simulink model "allmodes"  (Simulink 7.4)
settings: Solver=ode23tb  StartTime=0.0  StopTime=inf  MaxStep=1e-4  RelTol=1e-4
undefined symbols (not defined in the file): Ion, Lithium
libraries: powerlib x185, electricdrivelib x21, powerlib_extras x19, simulink x5
(part 2 of 7)

== system allmodes/battery controller /SUIM1 ==
  Ibref-SUIM : Inport
  Add : Sum  OutDataType=fixdt(1, 16)  OutScaling=2^-10
  Add1 : Sum  Inputs=+-  OutDataType=fixdt(1, 16)  OutScaling=2^-10
  Gain1 : Gain  Gain=0.025  ParameterDataType=fixdt(1, 16)  ParameterScaling=2^0  OutDataType=fixdt(1, 16)  OutScaling=2^0
  Gain2 : Gain  Gain=0.8  ParameterDataType=fixdt(1, 16)  ParameterScaling=2^0  OutDataType=fixdt(1, 16)  OutScaling=2^0
  Integrator : Integrator
  Memory : Memory  X0=200
  Saturation : Saturate  UpperLimit=1  LowerLimit=-1  OutDataType=fixdt(1, 16)  OutScaling=2^0
  Saturation1 : Saturate  UpperLimit=1.01  LowerLimit=0.1  OutDataType=fixdt(1, 16)  OutScaling=2^0
  Subsystem : Subsystem
  Subsystem1 : Subsystem
  Subsystem2 : Subsystem
  Subsystem3 : Subsystem
  Sum : Sum  Inputs=|++  OutDataType=fixdt(1, 16)  OutScaling=2^0
  Sum10 : Sum  Inputs=++|  OutDataType=fixdt(1, 16)  OutScaling=2^0
  Sum2 : Sum  Inputs=|++  OutDataType=fixdt(1, 16)  OutScaling=2^0
  Sum{3..4,7..8} (4 alike) : Sum  Inputs=|+-  OutDataType=fixdt(1, 16)  OutScaling=2^0
  Sum5 : Sum  Inputs=|++  OutDataType=fixdt(1, 16)  OutScaling=2^0
  Sum6 : Sum  Inputs=+|+|+  OutDataType=fixdt(1, 16)  OutScaling=2^0
  Sum9 : Sum  Inputs=|+-+  OutDataType=fixdt(1, 16)  OutScaling=2^0
  Switch : Switch  Threshold=400*0.3  OutDataType=fixdt(1, 16)  OutScaling=2^0
  Switch1 : Switch  Threshold=99.999999  OutDataType=fixdt(1, 16)  OutScaling=2^0
  Switch2 : Switch  Threshold=99.999999  OutDataType=fixdt(1, 16)  OutScaling=2^0
  Transfer Fcn1 : TransferFcn  Numerator=1  Denominator=[1/(10) 1]
  Transport Delay : TransportDelay  DelayTime=2
  Transport Delay1 : TransportDelay  DelayTime=2
  ain1 : Gain  Gain=0.25  ParameterDataType=fixdt(1, 16)  ParameterScaling=2^0  OutDataType=fixdt(1, 16)  OutScaling=2^0
  ain2 : Gain  Gain=1/700  ParameterDataType=fixdt(1, 16)  ParameterScaling=2^0  OutDataType=fixdt(1, 16)  OutScaling=2^0
  ain3 : Gain  Gain=1/16.5  ParameterDataType=fixdt(1, 16)  ParameterScaling=2^0  OutDataType=fixdt(1, 16)  OutScaling=2^0
  ain4 : Gain  Gain=700  ParameterDataType=fixdt(1, 16)  ParameterScaling=2^0  OutDataType=fixdt(1, 16)  OutScaling=2^0
  ain5 : Gain  Gain=0.75  ParameterDataType=fixdt(1, 16)  ParameterScaling=2^0  OutDataType=fixdt(1, 16)  OutScaling=2^0
  ain6 : Gain  Gain=16.5  ParameterDataType=fixdt(1, 16)  ParameterScaling=2^0  OutDataType=fixdt(1, 16)  OutScaling=2^0
  ain7 : Gain  Gain=0.03  ParameterDataType=fixdt(1, 16)  ParameterScaling=2^0  OutDataType=fixdt(1, 16)  OutScaling=2^0
  ain8 : Gain  Gain=7  ParameterDataType=fixdt(1, 16)  ParameterScaling=2^0  OutDataType=fixdt(1, 16)  OutScaling=2^0
  ain9 : Gain  Gain=0.3  ParameterDataType=fixdt(1, 16)  ParameterScaling=2^0  OutDataType=fixdt(1, 16)  OutScaling=2^0
  tag scope: Ibrefs=global, boost=global, buck=global
  wires:
  Sum4/1 -> ain1/1, Subsystem2/1(In1)
  ain2/1 -> Saturation/1
  Subsystem2/1(Out1) -> Sum2/1
  ain1/1 -> Sum2/2
  Saturation/1 -> ain4/1, Switch1/3
  ain4/1 -> Sum3/1
  Sum3/1 -> ain3/1
  Subsystem1/1(Out1) -> Sum6/2
  ain5/1 -> Sum6/3
  Sum7/1 -> ain5/1, Subsystem1/1(In1)
  Sum2/1 -> Sum5/1
  Sum5/1 -> Sum8/1
  Sum8/1 -> ain6/1, Sum10/2
  Subsystem3/1(Out1) -> Sum/1
  ain6/1 -> Sum/2
  Sum/1 -> Sum9/1
  Sum9/1 -> Sum3/2, ain2/1
  ain3/1 -> Sum10/1
  ain7/1 -> Sum9/2
  Sum6/1 -> Sum4/1
  Sum10/1 -> Subsystem3/1(In1)
  [VcSUIM] -> Sum4/2
  [VcSUIM] -> Sum9/3
  [IbSUIM] -> Sum7/2
  [IbSUIM] -> Sum5/2
  [VbSUIM] -> Sum6/1
  [ISUIM] -> ain7/1
  [ISUIM] -> Sum8/2
  Subsystem/2(Out2) -> [boost]
  Subsystem/1(Out1) -> [buck]
  Transfer Fcn1/1 -> Sum7/1, [Ibrefs]
  [ts] -> Subsystem/Enable
  [VbSUIM] -> Switch/2
  ain8/1 -> Switch/1
  ain9/1 -> Switch/3
  Ibref-SUIM/1 -> ain8/1, ain9/1
  Switch/1 -> Transfer Fcn1/1
  [VbSUIM] -> Add1/2
  Add1/1 -> Gain1/1, Gain2/1
  [VbSUIM] -> Switch2/3
  [soc] -> Transport Delay1/1
  Transport Delay1/1 -> Switch2/2
  Add/1 -> Saturation1/1
  Gain1/1 -> Add/2
  Integrator/1 -> Add/1
  Gain2/1 -> Integrator/1
  Switch2/1 -> Add1/1, Memory/1
  Memory/1 -> Switch2/1
  Switch1/1 -> Subsystem/1(In1)
  [soc] -> Transport Delay/1
  Saturation1/1 -> Switch1/1
  Transport Delay/1 -> Switch1/2

== system allmodes/battery controller /mode selector ==
  In1 : Inport
  Constant33 : Constant  Value=[0 1 0 0 0 0 0 0 0 0 0 0 0 0 0 0 0 0 0 0 0]  OutDataType=fixdt(1, 16)  OutScaling=2^0
  Constant34 : Constant  Value=[0 1 1 1 1 0 0 0 0 0 0 0 0 0 0 0 0 0 0 0 0]  OutDataType=fixdt(1, 16)  OutScaling=2^0
  Constant35 : Constant  Value=[0 1 1 1 1 1 1 0 0 0 0 0 0 0 0 0 0 0 0 0 0]  OutDataType=fixdt(1, 16)  OutScaling=2^0
  Constant36 : Constant  Value=[0 1 1 1 1 1 1 1 1 1 1 1 1 0 0 0 0 0 0 0 0]  OutDataType=fixdt(1, 16)  OutScaling=2^0
  Constant37 : Constant  Value=[0 1 1 1 1 1 1 1 1 1 1 1 1 1 1 1 1 1 1 1 1]  OutDataType=fixdt(1, 16)  OutScaling=2^0
  Constant38 : Constant  Value=[0 1 1 0 0 0 0 0 0 0 0 0 0 0 0 0 0 0 0 0 0]  OutDataType=fixdt(1, 16)  OutScaling=2^0
  Constant39 : Constant  Value=[0 1 1 1 1 0 0 0 0 0 0 0 0 0 0 0 0 0 0 0 0]  OutDataType=fixdt(1, 16)  OutScaling=2^0
  Constant40 : Constant  Value=[0 1 1 1 1 1 1 1 1 0 0 0 0 0 0 0 0 0 0 0 0]  OutDataType=fixdt(1, 16)  OutScaling=2^0
  Constant41 : Constant  Value=[0 1 1 1 1 1 1 1 1 1 1 1 1 1 1 1 1 0 0 0 0]  OutDataType=fixdt(1, 16)  OutScaling=2^0
  Constant42 : Constant  Value=[0 1 1 1 1 1 1 1 1 1 1 0 0 0 0 0 0 0 0 0 0]  OutDataType=fixdt(1, 16)  OutScaling=2^0
  Constant43 : Constant  Value=[1 1 1 1 1 1 1 1 1 1 1 1 1 1 1 1 1 1 1 1 1]  OutDataType=fixdt(1, 16)  OutScaling=2^0
  Constant44 : Constant  Value=[0 1 1 0 0 0 0 0 0 0 0 0 0 0 0 0 0 0 0 0 0]  OutDataType=fixdt(1, 16)  OutScaling=2^0
  Constant45 : Constant  Value=[0 1 1 1 1 1 1 1 1 1 1 1 1 1 1 1 1 1 1 1 1]  OutDataType=fixdt(1, 16)  OutScaling=2^0
  Constant46 : Constant  Value=[0 1 1 1 1 1 1 1 1 1 1 0 0 0 0 0 0 0 0 0 0]  OutDataType=fixdt(1, 16)  OutScaling=2^0
  Constant47 : Constant  Value=[0 1 1 1 1 1 1 1 1 1 1 0 0 0 0 0 0 0 0 0 0]  OutDataType=fixdt(1, 16)  OutScaling=2^0
  Constant48 : Constant  Value=[0 1 1 1 1 1 1 1 1 1 1 1 1 1 1 1 1 1 1 1 1]  OutDataType=fixdt(1, 16)  OutScaling=2^0
  Constant{49..52} (4 alike) : Constant  Value=[1 0 0 0 0 0 0 0 0 0 0 0 0 0 0 0 0 0 0 0 0]  OutDataType=fixdt(1, 16)  OutScaling=2^0
  Constant53 : Constant  Value=[0 1 0 0 0 0 0 0 0 0 0 0 0 0 0 0 0 0 0 0 0]  OutDataType=fixdt(1, 16)  OutScaling=2^0
  Demux : Demux  Outputs=21
  Multiport Switch : MultiPortSwitch  Inputs=21  OutDataType=fixdt(1, 16)  OutScaling=2^0
  tag scope: ts=global, tv10=global, tv11=global, tv12=global, tv13=global, tv14=global, tv15=global, tv16=global, tv17=global, tv18=global, tv19=global, tv1=global, tv20=global, tv2=global, tv3=global, tv4=global, tv5=global, tv6=global, tv7=global, tv8=global, tv9=global
  wires:
  Constant33/1 -> Multiport Switch/2
  Constant44/1 -> Multiport Switch/3
  Constant47/1 -> Multiport Switch/4
  Constant48/1 -> Multiport Switch/5
  Constant49/1 -> Multiport Switch/6
  Constant50/1 -> Multiport Switch/7
  Constant51/1 -> Multiport Switch/8
  Constant52/1 -> Multiport Switch/9
  Constant53/1 -> Multiport Switch/10
  Constant34/1 -> Multiport Switch/11
  Constant35/1 -> Multiport Switch/12
  Constant36/1 -> Multiport Switch/13
  Constant37/1 -> Multiport Switch/14
  Multiport Switch/1 -> Demux/1
  Constant38/1 -> Multiport Switch/15
  Constant39/1 -> Multiport Switch/16
  Constant40/1 -> Multiport Switch/17
  Constant41/1 -> Multiport Switch/18
  Constant42/1 -> Multiport Switch/19
  Constant43/1 -> Multiport Switch/22
  Constant45/1 -> Multiport Switch/21
  Constant46/1 -> Multiport Switch/20
  Demux/1 -> [ts]
  Demux/2 -> [tv1]
  Demux/3 -> [tv2]
  Demux/4 -> [tv3]
  Demux/5 -> [tv4]
  Demux/6 -> [tv5]
  Demux/7 -> [tv6]
  Demux/8 -> [tv7]
  Demux/9 -> [tv8]
  Demux/10 -> [tv9]
  Demux/11 -> [tv10]
  Demux/12 -> [tv11]
  Demux/13 -> [tv12]
  Demux/14 -> [tv13]
  Demux/15 -> [tv14]
  Demux/16 -> [tv15]
  Demux/17 -> [tv16]
  Demux/18 -> [tv17]
  Demux/19 -> [tv18]
  Demux/20 -> [tv19]
  Demux/21 -> [tv20]
  In1/1 -> Multiport Switch/1

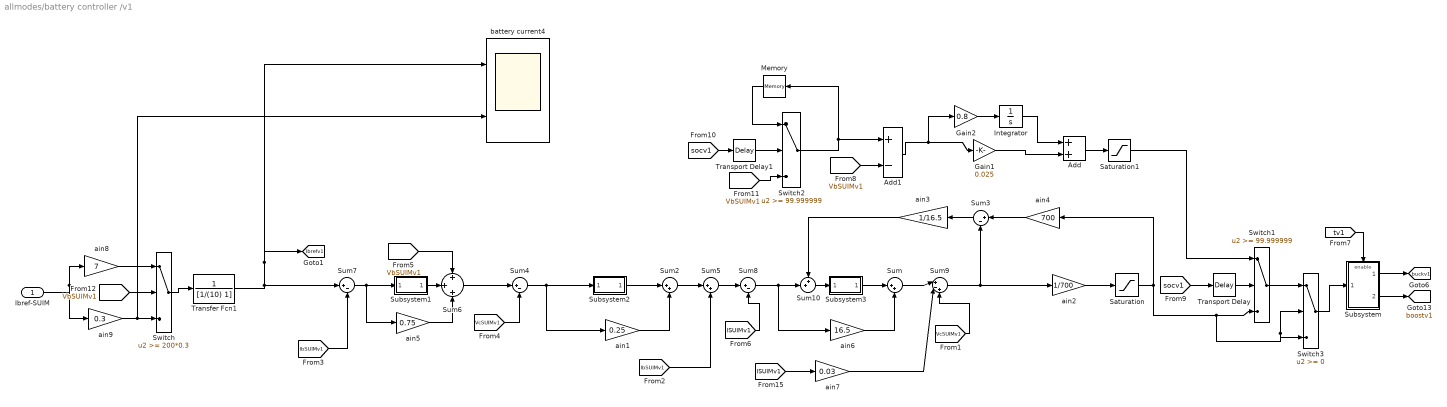
== system allmodes/battery controller /v1 ==
  Ibref-SUIM : Inport
  Add : Sum  OutDataType=fixdt(1, 16)  OutScaling=2^-10
  Add1 : Sum  Inputs=+-  OutDataType=fixdt(1, 16)  OutScaling=2^-10
  Gain1 : Gain  Gain=0.025  ParameterDataType=fixdt(1, 16)  ParameterScaling=2^0  OutDataType=fixdt(1, 16)  OutScaling=2^0
  Gain2 : Gain  Gain=0.8  ParameterDataType=fixdt(1, 16)  ParameterScaling=2^0  OutDataType=fixdt(1, 16)  OutScaling=2^0
  Integrator : Integrator
  Memory : Memory  X0=200
  Saturation : Saturate  UpperLimit=1  LowerLimit=-1  OutDataType=fixdt(1, 16)  OutScaling=2^0
  Saturation1 : Saturate  UpperLimit=1.01  LowerLimit=0.1  OutDataType=fixdt(1, 16)  OutScaling=2^0
  Subsystem : Subsystem
  Subsystem1 : Subsystem
  Subsystem2 : Subsystem
  Subsystem3 : Subsystem
  Sum : Sum  Inputs=|++  OutDataType=fixdt(1, 16)  OutScaling=2^0
  Sum10 : Sum  Inputs=++|  OutDataType=fixdt(1, 16)  OutScaling=2^0
  Sum2 : Sum  Inputs=|++  OutDataType=fixdt(1, 16)  OutScaling=2^0
  Sum{3..4,7..8} (4 alike) : Sum  Inputs=|+-  OutDataType=fixdt(1, 16)  OutScaling=2^0
  Sum5 : Sum  Inputs=|++  OutDataType=fixdt(1, 16)  OutScaling=2^0
  Sum6 : Sum  Inputs=+|+|+  OutDataType=fixdt(1, 16)  OutScaling=2^0
  Sum9 : Sum  Inputs=|+-+  OutDataType=fixdt(1, 16)  OutScaling=2^0
  Switch : Switch  Threshold=200*0.3  OutDataType=fixdt(1, 16)  OutScaling=2^0
  Switch1 : Switch  Threshold=99.999999  OutDataType=fixdt(1, 16)  OutScaling=2^0
  Switch2 : Switch  Threshold=99.999999  OutDataType=fixdt(1, 16)  OutScaling=2^0
  Switch3 : Switch  OutDataType=fixdt(1, 16)  OutScaling=2^0
  Transfer Fcn1 : TransferFcn  Numerator=1  Denominator=[1/(10) 1]
  Transport Delay : TransportDelay  DelayTime=2
  Transport Delay1 : TransportDelay  DelayTime=2
  ain1 : Gain  Gain=0.25  ParameterDataType=fixdt(1, 16)  ParameterScaling=2^0  OutDataType=fixdt(1, 16)  OutScaling=2^0
  ain2 : Gain  Gain=1/700  ParameterDataType=fixdt(1, 16)  ParameterScaling=2^0  OutDataType=fixdt(1, 16)  OutScaling=2^0
  ain3 : Gain  Gain=1/16.5  ParameterDataType=fixdt(1, 16)  ParameterScaling=2^0  OutDataType=fixdt(1, 16)  OutScaling=2^0
  ain4 : Gain  Gain=700  ParameterDataType=fixdt(1, 16)  ParameterScaling=2^0  OutDataType=fixdt(1, 16)  OutScaling=2^0
  ain5 : Gain  Gain=0.75  ParameterDataType=fixdt(1, 16)  ParameterScaling=2^0  OutDataType=fixdt(1, 16)  OutScaling=2^0
  ain6 : Gain  Gain=16.5  ParameterDataType=fixdt(1, 16)  ParameterScaling=2^0  OutDataType=fixdt(1, 16)  OutScaling=2^0
  ain7 : Gain  Gain=0.03  ParameterDataType=fixdt(1, 16)  ParameterScaling=2^0  OutDataType=fixdt(1, 16)  OutScaling=2^0
  ain8 : Gain  Gain=7  ParameterDataType=fixdt(1, 16)  ParameterScaling=2^0  OutDataType=fixdt(1, 16)  OutScaling=2^0
  ain9 : Gain  Gain=0.3  ParameterDataType=fixdt(1, 16)  ParameterScaling=2^0  OutDataType=fixdt(1, 16)  OutScaling=2^0
  battery current4 : Scope  NumInputPorts=2
      settings: TimeRange=0.25  YMin=460~30  YMax=660~30  SaveName=ScopeData7
  tag scope: Ibrefv1=global, boostv1=global, buckv1=global
  wires:
  Transfer Fcn1/1 -> Sum7/1, [Ibrefv1], battery current4/1
  Subsystem/1(Out1) -> [buckv1]
  Subsystem/2(Out2) -> [boostv1]
  [ISUIMv1] -> Sum8/2
  [ISUIMv1] -> ain7/1
  [VbSUIMv1] -> Sum6/1
  [IbSUIMv1] -> Sum5/2
  [IbSUIMv1] -> Sum7/2
  [VcSUIMv1] -> Sum9/3
  [VcSUIMv1] -> Sum4/2
  Sum10/1 -> Subsystem3/1(In1)
  Sum6/1 -> Sum4/1
  ain7/1 -> Sum9/2
  ain3/1 -> Sum10/1
  Sum9/1 -> ain2/1, Sum3/2
  Sum/1 -> Sum9/1
  ain6/1 -> Sum/2
  Subsystem3/1(Out1) -> Sum/1
  Sum8/1 -> Sum10/2, ain6/1
  Sum5/1 -> Sum8/1
  Sum2/1 -> Sum5/1
  Sum7/1 -> Subsystem1/1(In1), ain5/1
  ain5/1 -> Sum6/3
  Subsystem1/1(Out1) -> Sum6/2
  Sum3/1 -> ain3/1
  ain4/1 -> Sum3/1
  Saturation/1 -> ain4/1, Switch1/3, Switch3/3, Switch3/2
  ain1/1 -> Sum2/2
  Subsystem2/1(Out1) -> Sum2/1
  ain2/1 -> Saturation/1
  Sum4/1 -> Subsystem2/1(In1), ain1/1
  [tv1] -> Subsystem/Enable
  [VbSUIMv1] -> Add1/2
  Add1/1 -> Gain1/1, Gain2/1
  [VbSUIMv1] -> Switch2/3
  [socv1] -> Transport Delay1/1
  Transport Delay1/1 -> Switch2/2
  Add/1 -> Saturation1/1
  Gain1/1 -> Add/2
  Integrator/1 -> Add/1
  Gain2/1 -> Integrator/1
  Switch2/1 -> Add1/1, Memory/1
  Memory/1 -> Switch2/1
  [socv1] -> Transport Delay/1
  Transport Delay/1 -> Switch1/2
  Saturation1/1 -> Switch1/1
  [VbSUIMv1] -> Switch/2
  ain8/1 -> Switch/1
  ain9/1 -> Switch/3, battery current4/2
  Switch/1 -> Transfer Fcn1/1
  Ibref-SUIM/1 -> ain8/1, ain9/1
  Switch1/1 -> Switch3/1
  Switch3/1 -> Subsystem/1(In1)

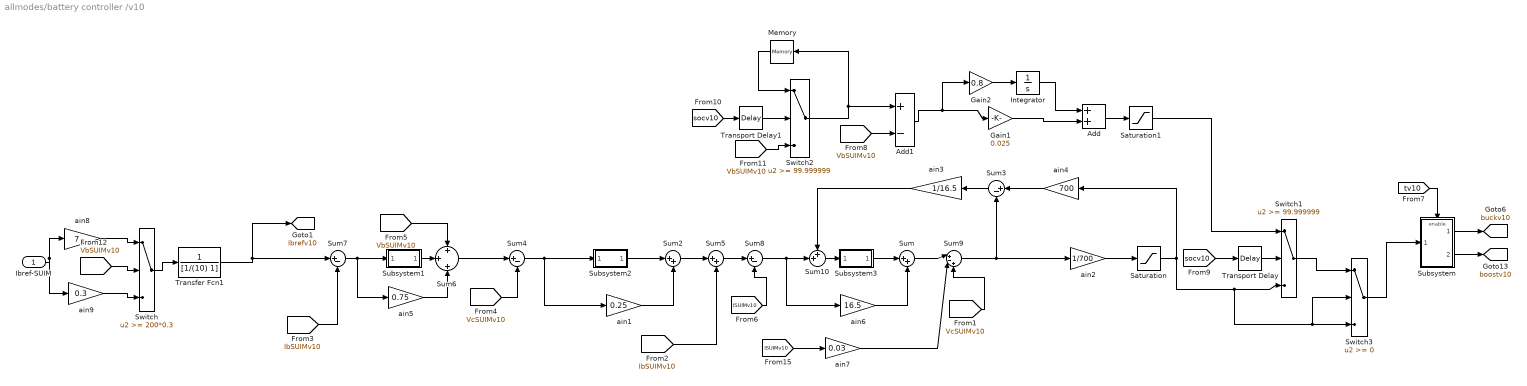
== system allmodes/battery controller /v10 ==
  Ibref-SUIM : Inport
  Add : Sum  OutDataType=fixdt(1, 16)  OutScaling=2^-10
  Add1 : Sum  Inputs=+-  OutDataType=fixdt(1, 16)  OutScaling=2^-10
  Gain1 : Gain  Gain=0.025  ParameterDataType=fixdt(1, 16)  ParameterScaling=2^0  OutDataType=fixdt(1, 16)  OutScaling=2^0
  Gain2 : Gain  Gain=0.8  ParameterDataType=fixdt(1, 16)  ParameterScaling=2^0  OutDataType=fixdt(1, 16)  OutScaling=2^0
  Integrator : Integrator
  Memory : Memory  X0=200
  Saturation : Saturate  UpperLimit=1  LowerLimit=-1  OutDataType=fixdt(1, 16)  OutScaling=2^0
  Saturation1 : Saturate  UpperLimit=1.01  LowerLimit=0.1  OutDataType=fixdt(1, 16)  OutScaling=2^0
  Subsystem : Subsystem
  Subsystem1 : Subsystem
  Subsystem2 : Subsystem
  Subsystem3 : Subsystem
  Sum : Sum  Inputs=|++  OutDataType=fixdt(1, 16)  OutScaling=2^0
  Sum10 : Sum  Inputs=++|  OutDataType=fixdt(1, 16)  OutScaling=2^0
  Sum2 : Sum  Inputs=|++  OutDataType=fixdt(1, 16)  OutScaling=2^0
  Sum{3..4,7..8} (4 alike) : Sum  Inputs=|+-  OutDataType=fixdt(1, 16)  OutScaling=2^0
  Sum5 : Sum  Inputs=|++  OutDataType=fixdt(1, 16)  OutScaling=2^0
  Sum6 : Sum  Inputs=+|+|+  OutDataType=fixdt(1, 16)  OutScaling=2^0
  Sum9 : Sum  Inputs=|+-+  OutDataType=fixdt(1, 16)  OutScaling=2^0
  Switch : Switch  Threshold=200*0.3  OutDataType=fixdt(1, 16)  OutScaling=2^0
  Switch1 : Switch  Threshold=99.999999  OutDataType=fixdt(1, 16)  OutScaling=2^0
  Switch2 : Switch  Threshold=99.999999  OutDataType=fixdt(1, 16)  OutScaling=2^0
  Switch3 : Switch  OutDataType=fixdt(1, 16)  OutScaling=2^0
  Transfer Fcn1 : TransferFcn  Numerator=1  Denominator=[1/(10) 1]
  Transport Delay : TransportDelay  DelayTime=2
  Transport Delay1 : TransportDelay  DelayTime=2
  ain1 : Gain  Gain=0.25  ParameterDataType=fixdt(1, 16)  ParameterScaling=2^0  OutDataType=fixdt(1, 16)  OutScaling=2^0
  ain2 : Gain  Gain=1/700  ParameterDataType=fixdt(1, 16)  ParameterScaling=2^0  OutDataType=fixdt(1, 16)  OutScaling=2^0
  ain3 : Gain  Gain=1/16.5  ParameterDataType=fixdt(1, 16)  ParameterScaling=2^0  OutDataType=fixdt(1, 16)  OutScaling=2^0
  ain4 : Gain  Gain=700  ParameterDataType=fixdt(1, 16)  ParameterScaling=2^0  OutDataType=fixdt(1, 16)  OutScaling=2^0
  ain5 : Gain  Gain=0.75  ParameterDataType=fixdt(1, 16)  ParameterScaling=2^0  OutDataType=fixdt(1, 16)  OutScaling=2^0
  ain6 : Gain  Gain=16.5  ParameterDataType=fixdt(1, 16)  ParameterScaling=2^0  OutDataType=fixdt(1, 16)  OutScaling=2^0
  ain7 : Gain  Gain=0.03  ParameterDataType=fixdt(1, 16)  ParameterScaling=2^0  OutDataType=fixdt(1, 16)  OutScaling=2^0
  ain8 : Gain  Gain=7  ParameterDataType=fixdt(1, 16)  ParameterScaling=2^0  OutDataType=fixdt(1, 16)  OutScaling=2^0
  ain9 : Gain  Gain=0.3  ParameterDataType=fixdt(1, 16)  ParameterScaling=2^0  OutDataType=fixdt(1, 16)  OutScaling=2^0
  tag scope: Ibrefv10=global, boostv10=global, buckv10=global
  wires:
  Ibref-SUIM/1 -> ain9/1, ain8/1
  Switch/1 -> Transfer Fcn1/1
  ain9/1 -> Switch/3
  ain8/1 -> Switch/1
  [VbSUIMv10] -> Switch/2
  Saturation1/1 -> Switch1/1
  Transport Delay/1 -> Switch1/2
  [socv10] -> Transport Delay/1
  Memory/1 -> Switch2/1
  Switch2/1 -> Memory/1, Add1/1
  Gain2/1 -> Integrator/1
  Integrator/1 -> Add/1
  Gain1/1 -> Add/2
  Add/1 -> Saturation1/1
  Transport Delay1/1 -> Switch2/2
  [socv10] -> Transport Delay1/1
  [VbSUIMv10] -> Switch2/3
  Add1/1 -> Gain2/1, Gain1/1
  [VbSUIMv10] -> Add1/2
  [tv10] -> Subsystem/Enable
  Sum4/1 -> ain1/1, Subsystem2/1(In1)
  ain2/1 -> Saturation/1
  Subsystem2/1(Out1) -> Sum2/1
  ain1/1 -> Sum2/2
  Saturation/1 -> ain4/1, Switch1/3, Switch3/3, Switch3/2
  ain4/1 -> Sum3/1
  Sum3/1 -> ain3/1
  Subsystem1/1(Out1) -> Sum6/2
  ain5/1 -> Sum6/3
  Sum7/1 -> ain5/1, Subsystem1/1(In1)
  Sum2/1 -> Sum5/1
  Sum5/1 -> Sum8/1
  Sum8/1 -> ain6/1, Sum10/2
  Subsystem3/1(Out1) -> Sum/1
  ain6/1 -> Sum/2
  Sum/1 -> Sum9/1
  Sum9/1 -> Sum3/2, ain2/1
  ain3/1 -> Sum10/1
  ain7/1 -> Sum9/2
  Sum6/1 -> Sum4/1
  Sum10/1 -> Subsystem3/1(In1)
  [VcSUIMv10] -> Sum4/2
  [VcSUIMv10] -> Sum9/3
  [IbSUIMv10] -> Sum7/2
  [IbSUIMv10] -> Sum5/2
  [VbSUIMv10] -> Sum6/1
  [ISUIMv10] -> ain7/1
  [ISUIMv10] -> Sum8/2
  Subsystem/2(Out2) -> [boostv10]
  Subsystem/1(Out1) -> [buckv10]
  Transfer Fcn1/1 -> [Ibrefv10], Sum7/1
  Switch1/1 -> Switch3/1
  Switch3/1 -> Subsystem/1(In1)

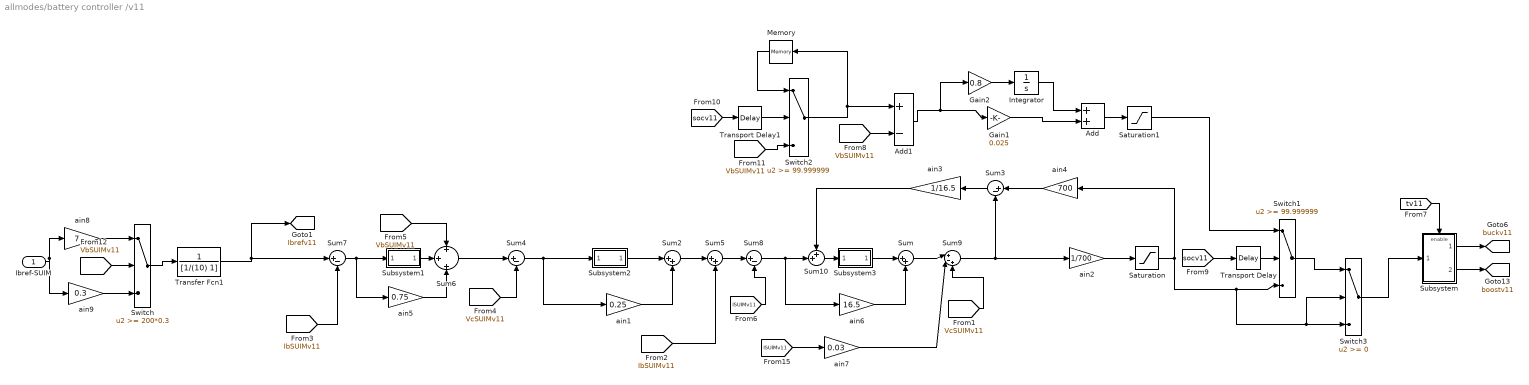
== system allmodes/battery controller /v11 ==
  Ibref-SUIM : Inport
  Add : Sum  OutDataType=fixdt(1, 16)  OutScaling=2^-10
  Add1 : Sum  Inputs=+-  OutDataType=fixdt(1, 16)  OutScaling=2^-10
  Gain1 : Gain  Gain=0.025  ParameterDataType=fixdt(1, 16)  ParameterScaling=2^0  OutDataType=fixdt(1, 16)  OutScaling=2^0
  Gain2 : Gain  Gain=0.8  ParameterDataType=fixdt(1, 16)  ParameterScaling=2^0  OutDataType=fixdt(1, 16)  OutScaling=2^0
  Integrator : Integrator
  Memory : Memory  X0=200
  Saturation : Saturate  UpperLimit=1  LowerLimit=-1  OutDataType=fixdt(1, 16)  OutScaling=2^0
  Saturation1 : Saturate  UpperLimit=1.01  LowerLimit=0.1  OutDataType=fixdt(1, 16)  OutScaling=2^0
  Subsystem : Subsystem
  Subsystem1 : Subsystem
  Subsystem2 : Subsystem
  Subsystem3 : Subsystem
  Sum : Sum  Inputs=|++  OutDataType=fixdt(1, 16)  OutScaling=2^0
  Sum10 : Sum  Inputs=++|  OutDataType=fixdt(1, 16)  OutScaling=2^0
  Sum2 : Sum  Inputs=|++  OutDataType=fixdt(1, 16)  OutScaling=2^0
  Sum{3..4,7..8} (4 alike) : Sum  Inputs=|+-  OutDataType=fixdt(1, 16)  OutScaling=2^0
  Sum5 : Sum  Inputs=|++  OutDataType=fixdt(1, 16)  OutScaling=2^0
  Sum6 : Sum  Inputs=+|+|+  OutDataType=fixdt(1, 16)  OutScaling=2^0
  Sum9 : Sum  Inputs=|+-+  OutDataType=fixdt(1, 16)  OutScaling=2^0
  Switch : Switch  Threshold=200*0.3  OutDataType=fixdt(1, 16)  OutScaling=2^0
  Switch1 : Switch  Threshold=99.999999  OutDataType=fixdt(1, 16)  OutScaling=2^0
  Switch2 : Switch  Threshold=99.999999  OutDataType=fixdt(1, 16)  OutScaling=2^0
  Switch3 : Switch  OutDataType=fixdt(1, 16)  OutScaling=2^0
  Transfer Fcn1 : TransferFcn  Numerator=1  Denominator=[1/(10) 1]
  Transport Delay : TransportDelay  DelayTime=2
  Transport Delay1 : TransportDelay  DelayTime=2
  ain1 : Gain  Gain=0.25  ParameterDataType=fixdt(1, 16)  ParameterScaling=2^0  OutDataType=fixdt(1, 16)  OutScaling=2^0
  ain2 : Gain  Gain=1/700  ParameterDataType=fixdt(1, 16)  ParameterScaling=2^0  OutDataType=fixdt(1, 16)  OutScaling=2^0
  ain3 : Gain  Gain=1/16.5  ParameterDataType=fixdt(1, 16)  ParameterScaling=2^0  OutDataType=fixdt(1, 16)  OutScaling=2^0
  ain4 : Gain  Gain=700  ParameterDataType=fixdt(1, 16)  ParameterScaling=2^0  OutDataType=fixdt(1, 16)  OutScaling=2^0
  ain5 : Gain  Gain=0.75  ParameterDataType=fixdt(1, 16)  ParameterScaling=2^0  OutDataType=fixdt(1, 16)  OutScaling=2^0
  ain6 : Gain  Gain=16.5  ParameterDataType=fixdt(1, 16)  ParameterScaling=2^0  OutDataType=fixdt(1, 16)  OutScaling=2^0
  ain7 : Gain  Gain=0.03  ParameterDataType=fixdt(1, 16)  ParameterScaling=2^0  OutDataType=fixdt(1, 16)  OutScaling=2^0
  ain8 : Gain  Gain=7  ParameterDataType=fixdt(1, 16)  ParameterScaling=2^0  OutDataType=fixdt(1, 16)  OutScaling=2^0
  ain9 : Gain  Gain=0.3  ParameterDataType=fixdt(1, 16)  ParameterScaling=2^0  OutDataType=fixdt(1, 16)  OutScaling=2^0
  tag scope: Ibrefv11=global, boostv11=global, buckv11=global
  wires:
  Ibref-SUIM/1 -> ain9/1, ain8/1
  Switch/1 -> Transfer Fcn1/1
  ain9/1 -> Switch/3
  ain8/1 -> Switch/1
  [VbSUIMv11] -> Switch/2
  Saturation1/1 -> Switch1/1
  Transport Delay/1 -> Switch1/2
  [socv11] -> Transport Delay/1
  Memory/1 -> Switch2/1
  Switch2/1 -> Memory/1, Add1/1
  Gain2/1 -> Integrator/1
  Integrator/1 -> Add/1
  Gain1/1 -> Add/2
  Add/1 -> Saturation1/1
  Transport Delay1/1 -> Switch2/2
  [socv11] -> Transport Delay1/1
  [VbSUIMv11] -> Switch2/3
  Add1/1 -> Gain2/1, Gain1/1
  [VbSUIMv11] -> Add1/2
  [tv11] -> Subsystem/Enable
  Sum4/1 -> ain1/1, Subsystem2/1(In1)
  ain2/1 -> Saturation/1
  Subsystem2/1(Out1) -> Sum2/1
  ain1/1 -> Sum2/2
  Saturation/1 -> ain4/1, Switch1/3, Switch3/3, Switch3/2
  ain4/1 -> Sum3/1
  Sum3/1 -> ain3/1
  Subsystem1/1(Out1) -> Sum6/2
  ain5/1 -> Sum6/3
  Sum7/1 -> ain5/1, Subsystem1/1(In1)
  Sum2/1 -> Sum5/1
  Sum5/1 -> Sum8/1
  Sum8/1 -> ain6/1, Sum10/2
  Subsystem3/1(Out1) -> Sum/1
  ain6/1 -> Sum/2
  Sum/1 -> Sum9/1
  Sum9/1 -> Sum3/2, ain2/1
  ain3/1 -> Sum10/1
  ain7/1 -> Sum9/2
  Sum6/1 -> Sum4/1
  Sum10/1 -> Subsystem3/1(In1)
  [VcSUIMv11] -> Sum4/2
  [VcSUIMv11] -> Sum9/3
  [IbSUIMv11] -> Sum7/2
  [IbSUIMv11] -> Sum5/2
  [VbSUIMv11] -> Sum6/1
  [ISUIMv11] -> ain7/1
  [ISUIMv11] -> Sum8/2
  Subsystem/2(Out2) -> [boostv11]
  Subsystem/1(Out1) -> [buckv11]
  Transfer Fcn1/1 -> [Ibrefv11], Sum7/1
  Switch1/1 -> Switch3/1
  Switch3/1 -> Subsystem/1(In1)

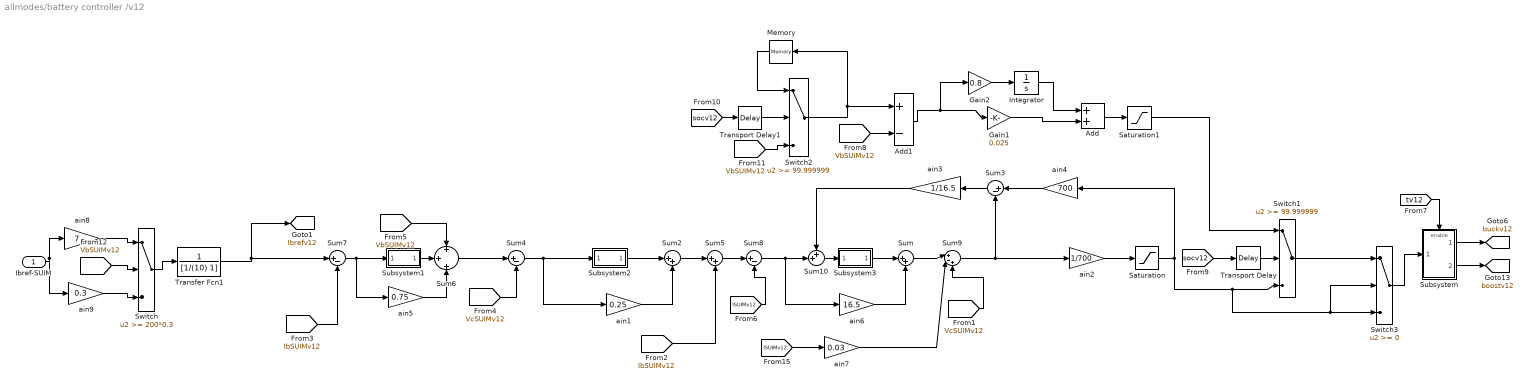
== system allmodes/battery controller /v12 ==
  Ibref-SUIM : Inport
  Add : Sum  OutDataType=fixdt(1, 16)  OutScaling=2^-10
  Add1 : Sum  Inputs=+-  OutDataType=fixdt(1, 16)  OutScaling=2^-10
  Gain1 : Gain  Gain=0.025  ParameterDataType=fixdt(1, 16)  ParameterScaling=2^0  OutDataType=fixdt(1, 16)  OutScaling=2^0
  Gain2 : Gain  Gain=0.8  ParameterDataType=fixdt(1, 16)  ParameterScaling=2^0  OutDataType=fixdt(1, 16)  OutScaling=2^0
  Integrator : Integrator
  Memory : Memory  X0=200
  Saturation : Saturate  UpperLimit=1  LowerLimit=-1  OutDataType=fixdt(1, 16)  OutScaling=2^0
  Saturation1 : Saturate  UpperLimit=1.01  LowerLimit=0.1  OutDataType=fixdt(1, 16)  OutScaling=2^0
  Subsystem : Subsystem
  Subsystem1 : Subsystem
  Subsystem2 : Subsystem
  Subsystem3 : Subsystem
  Sum : Sum  Inputs=|++  OutDataType=fixdt(1, 16)  OutScaling=2^0
  Sum10 : Sum  Inputs=++|  OutDataType=fixdt(1, 16)  OutScaling=2^0
  Sum2 : Sum  Inputs=|++  OutDataType=fixdt(1, 16)  OutScaling=2^0
  Sum{3..4,7..8} (4 alike) : Sum  Inputs=|+-  OutDataType=fixdt(1, 16)  OutScaling=2^0
  Sum5 : Sum  Inputs=|++  OutDataType=fixdt(1, 16)  OutScaling=2^0
  Sum6 : Sum  Inputs=+|+|+  OutDataType=fixdt(1, 16)  OutScaling=2^0
  Sum9 : Sum  Inputs=|+-+  OutDataType=fixdt(1, 16)  OutScaling=2^0
  Switch : Switch  Threshold=200*0.3  OutDataType=fixdt(1, 16)  OutScaling=2^0
  Switch1 : Switch  Threshold=99.999999  OutDataType=fixdt(1, 16)  OutScaling=2^0
  Switch2 : Switch  Threshold=99.999999  OutDataType=fixdt(1, 16)  OutScaling=2^0
  Switch3 : Switch  OutDataType=fixdt(1, 16)  OutScaling=2^0
  Transfer Fcn1 : TransferFcn  Numerator=1  Denominator=[1/(10) 1]
  Transport Delay : TransportDelay  DelayTime=2
  Transport Delay1 : TransportDelay  DelayTime=2
  ain1 : Gain  Gain=0.25  ParameterDataType=fixdt(1, 16)  ParameterScaling=2^0  OutDataType=fixdt(1, 16)  OutScaling=2^0
  ain2 : Gain  Gain=1/700  ParameterDataType=fixdt(1, 16)  ParameterScaling=2^0  OutDataType=fixdt(1, 16)  OutScaling=2^0
  ain3 : Gain  Gain=1/16.5  ParameterDataType=fixdt(1, 16)  ParameterScaling=2^0  OutDataType=fixdt(1, 16)  OutScaling=2^0
  ain4 : Gain  Gain=700  ParameterDataType=fixdt(1, 16)  ParameterScaling=2^0  OutDataType=fixdt(1, 16)  OutScaling=2^0
  ain5 : Gain  Gain=0.75  ParameterDataType=fixdt(1, 16)  ParameterScaling=2^0  OutDataType=fixdt(1, 16)  OutScaling=2^0
  ain6 : Gain  Gain=16.5  ParameterDataType=fixdt(1, 16)  ParameterScaling=2^0  OutDataType=fixdt(1, 16)  OutScaling=2^0
  ain7 : Gain  Gain=0.03  ParameterDataType=fixdt(1, 16)  ParameterScaling=2^0  OutDataType=fixdt(1, 16)  OutScaling=2^0
  ain8 : Gain  Gain=7  ParameterDataType=fixdt(1, 16)  ParameterScaling=2^0  OutDataType=fixdt(1, 16)  OutScaling=2^0
  ain9 : Gain  Gain=0.3  ParameterDataType=fixdt(1, 16)  ParameterScaling=2^0  OutDataType=fixdt(1, 16)  OutScaling=2^0
  tag scope: Ibrefv12=global, boostv12=global, buckv12=global
  wires:
  Ibref-SUIM/1 -> ain9/1, ain8/1
  Switch/1 -> Transfer Fcn1/1
  ain9/1 -> Switch/3
  ain8/1 -> Switch/1
  [VbSUIMv12] -> Switch/2
  Saturation1/1 -> Switch1/1
  Transport Delay/1 -> Switch1/2
  [socv12] -> Transport Delay/1
  Memory/1 -> Switch2/1
  Switch2/1 -> Memory/1, Add1/1
  Gain2/1 -> Integrator/1
  Integrator/1 -> Add/1
  Gain1/1 -> Add/2
  Add/1 -> Saturation1/1
  Transport Delay1/1 -> Switch2/2
  [socv12] -> Transport Delay1/1
  [VbSUIMv12] -> Switch2/3
  Add1/1 -> Gain2/1, Gain1/1
  [VbSUIMv12] -> Add1/2
  [tv12] -> Subsystem/Enable
  Sum4/1 -> ain1/1, Subsystem2/1(In1)
  ain2/1 -> Saturation/1
  Subsystem2/1(Out1) -> Sum2/1
  ain1/1 -> Sum2/2
  Saturation/1 -> ain4/1, Switch1/3, Switch3/3, Switch3/2
  ain4/1 -> Sum3/1
  Sum3/1 -> ain3/1
  Subsystem1/1(Out1) -> Sum6/2
  ain5/1 -> Sum6/3
  Sum7/1 -> ain5/1, Subsystem1/1(In1)
  Sum2/1 -> Sum5/1
  Sum5/1 -> Sum8/1
  Sum8/1 -> ain6/1, Sum10/2
  Subsystem3/1(Out1) -> Sum/1
  ain6/1 -> Sum/2
  Sum/1 -> Sum9/1
  Sum9/1 -> Sum3/2, ain2/1
  ain3/1 -> Sum10/1
  ain7/1 -> Sum9/2
  Sum6/1 -> Sum4/1
  Sum10/1 -> Subsystem3/1(In1)
  [VcSUIMv12] -> Sum4/2
  [VcSUIMv12] -> Sum9/3
  [IbSUIMv12] -> Sum7/2
  [IbSUIMv12] -> Sum5/2
  [VbSUIMv12] -> Sum6/1
  [ISUIMv12] -> ain7/1
  [ISUIMv12] -> Sum8/2
  Subsystem/2(Out2) -> [boostv12]
  Subsystem/1(Out1) -> [buckv12]
  Transfer Fcn1/1 -> [Ibrefv12], Sum7/1
  Switch1/1 -> Switch3/1
  Switch3/1 -> Subsystem/1(In1)

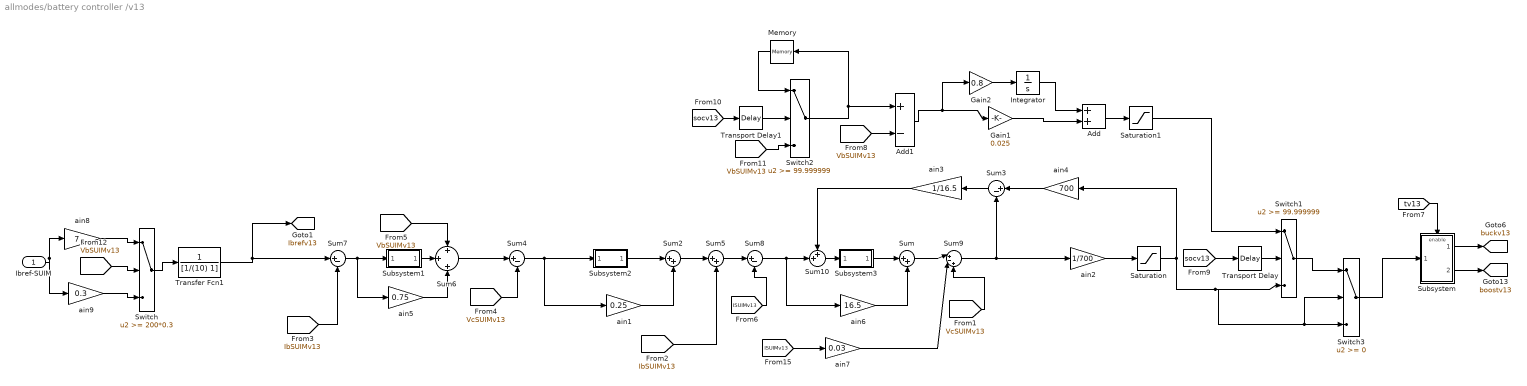
== system allmodes/battery controller /v13 ==
  Ibref-SUIM : Inport
  Add : Sum  OutDataType=fixdt(1, 16)  OutScaling=2^-10
  Add1 : Sum  Inputs=+-  OutDataType=fixdt(1, 16)  OutScaling=2^-10
  Gain1 : Gain  Gain=0.025  ParameterDataType=fixdt(1, 16)  ParameterScaling=2^0  OutDataType=fixdt(1, 16)  OutScaling=2^0
  Gain2 : Gain  Gain=0.8  ParameterDataType=fixdt(1, 16)  ParameterScaling=2^0  OutDataType=fixdt(1, 16)  OutScaling=2^0
  Integrator : Integrator
  Memory : Memory  X0=200
  Saturation : Saturate  UpperLimit=1  LowerLimit=-1  OutDataType=fixdt(1, 16)  OutScaling=2^0
  Saturation1 : Saturate  UpperLimit=1.01  LowerLimit=0.1  OutDataType=fixdt(1, 16)  OutScaling=2^0
  Subsystem : Subsystem
  Subsystem1 : Subsystem
  Subsystem2 : Subsystem
  Subsystem3 : Subsystem
  Sum : Sum  Inputs=|++  OutDataType=fixdt(1, 16)  OutScaling=2^0
  Sum10 : Sum  Inputs=++|  OutDataType=fixdt(1, 16)  OutScaling=2^0
  Sum2 : Sum  Inputs=|++  OutDataType=fixdt(1, 16)  OutScaling=2^0
  Sum{3..4,7..8} (4 alike) : Sum  Inputs=|+-  OutDataType=fixdt(1, 16)  OutScaling=2^0
  Sum5 : Sum  Inputs=|++  OutDataType=fixdt(1, 16)  OutScaling=2^0
  Sum6 : Sum  Inputs=+|+|+  OutDataType=fixdt(1, 16)  OutScaling=2^0
  Sum9 : Sum  Inputs=|+-+  OutDataType=fixdt(1, 16)  OutScaling=2^0
  Switch : Switch  Threshold=200*0.3  OutDataType=fixdt(1, 16)  OutScaling=2^0
  Switch1 : Switch  Threshold=99.999999  OutDataType=fixdt(1, 16)  OutScaling=2^0
  Switch2 : Switch  Threshold=99.999999  OutDataType=fixdt(1, 16)  OutScaling=2^0
  Switch3 : Switch  OutDataType=fixdt(1, 16)  OutScaling=2^0
  Transfer Fcn1 : TransferFcn  Numerator=1  Denominator=[1/(10) 1]
  Transport Delay : TransportDelay  DelayTime=2
  Transport Delay1 : TransportDelay  DelayTime=2
  ain1 : Gain  Gain=0.25  ParameterDataType=fixdt(1, 16)  ParameterScaling=2^0  OutDataType=fixdt(1, 16)  OutScaling=2^0
  ain2 : Gain  Gain=1/700  ParameterDataType=fixdt(1, 16)  ParameterScaling=2^0  OutDataType=fixdt(1, 16)  OutScaling=2^0
  ain3 : Gain  Gain=1/16.5  ParameterDataType=fixdt(1, 16)  ParameterScaling=2^0  OutDataType=fixdt(1, 16)  OutScaling=2^0
  ain4 : Gain  Gain=700  ParameterDataType=fixdt(1, 16)  ParameterScaling=2^0  OutDataType=fixdt(1, 16)  OutScaling=2^0
  ain5 : Gain  Gain=0.75  ParameterDataType=fixdt(1, 16)  ParameterScaling=2^0  OutDataType=fixdt(1, 16)  OutScaling=2^0
  ain6 : Gain  Gain=16.5  ParameterDataType=fixdt(1, 16)  ParameterScaling=2^0  OutDataType=fixdt(1, 16)  OutScaling=2^0
  ain7 : Gain  Gain=0.03  ParameterDataType=fixdt(1, 16)  ParameterScaling=2^0  OutDataType=fixdt(1, 16)  OutScaling=2^0
  ain8 : Gain  Gain=7  ParameterDataType=fixdt(1, 16)  ParameterScaling=2^0  OutDataType=fixdt(1, 16)  OutScaling=2^0
  ain9 : Gain  Gain=0.3  ParameterDataType=fixdt(1, 16)  ParameterScaling=2^0  OutDataType=fixdt(1, 16)  OutScaling=2^0
  tag scope: Ibrefv13=global, boostv13=global, buckv13=global
  wires:
  Ibref-SUIM/1 -> ain9/1, ain8/1
  Switch/1 -> Transfer Fcn1/1
  ain9/1 -> Switch/3
  ain8/1 -> Switch/1
  [VbSUIMv13] -> Switch/2
  Saturation1/1 -> Switch1/1
  Transport Delay/1 -> Switch1/2
  [socv13] -> Transport Delay/1
  Memory/1 -> Switch2/1
  Switch2/1 -> Memory/1, Add1/1
  Gain2/1 -> Integrator/1
  Integrator/1 -> Add/1
  Gain1/1 -> Add/2
  Add/1 -> Saturation1/1
  Transport Delay1/1 -> Switch2/2
  [socv13] -> Transport Delay1/1
  [VbSUIMv13] -> Switch2/3
  Add1/1 -> Gain2/1, Gain1/1
  [VbSUIMv13] -> Add1/2
  [tv13] -> Subsystem/Enable
  Sum4/1 -> ain1/1, Subsystem2/1(In1)
  ain2/1 -> Saturation/1
  Subsystem2/1(Out1) -> Sum2/1
  ain1/1 -> Sum2/2
  Saturation/1 -> ain4/1, Switch1/3, Switch3/3, Switch3/2
  ain4/1 -> Sum3/1
  Sum3/1 -> ain3/1
  Subsystem1/1(Out1) -> Sum6/2
  ain5/1 -> Sum6/3
  Sum7/1 -> ain5/1, Subsystem1/1(In1)
  Sum2/1 -> Sum5/1
  Sum5/1 -> Sum8/1
  Sum8/1 -> ain6/1, Sum10/2
  Subsystem3/1(Out1) -> Sum/1
  ain6/1 -> Sum/2
  Sum/1 -> Sum9/1
  Sum9/1 -> Sum3/2, ain2/1
  ain3/1 -> Sum10/1
  ain7/1 -> Sum9/2
  Sum6/1 -> Sum4/1
  Sum10/1 -> Subsystem3/1(In1)
  [VcSUIMv13] -> Sum4/2
  [VcSUIMv13] -> Sum9/3
  [IbSUIMv13] -> Sum7/2
  [IbSUIMv13] -> Sum5/2
  [VbSUIMv13] -> Sum6/1
  [ISUIMv13] -> ain7/1
  [ISUIMv13] -> Sum8/2
  Subsystem/2(Out2) -> [boostv13]
  Subsystem/1(Out1) -> [buckv13]
  Transfer Fcn1/1 -> [Ibrefv13], Sum7/1
  Switch1/1 -> Switch3/1
  Switch3/1 -> Subsystem/1(In1)

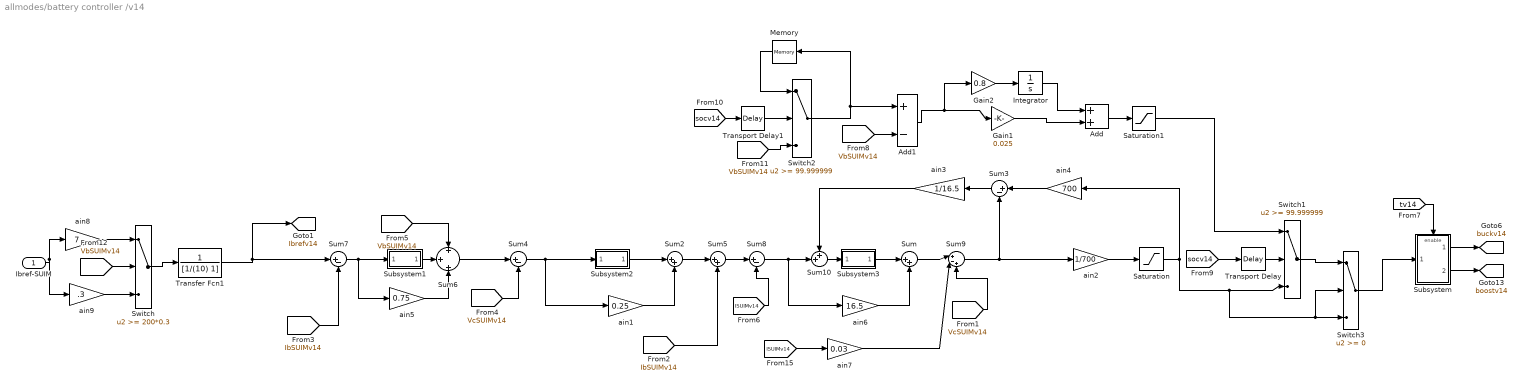
== system allmodes/battery controller /v14 ==
  Ibref-SUIM : Inport
  Add : Sum  OutDataType=fixdt(1, 16)  OutScaling=2^-10
  Add1 : Sum  Inputs=+-  OutDataType=fixdt(1, 16)  OutScaling=2^-10
  Gain1 : Gain  Gain=0.025  ParameterDataType=fixdt(1, 16)  ParameterScaling=2^0  OutDataType=fixdt(1, 16)  OutScaling=2^0
  Gain2 : Gain  Gain=0.8  ParameterDataType=fixdt(1, 16)  ParameterScaling=2^0  OutDataType=fixdt(1, 16)  OutScaling=2^0
  Integrator : Integrator
  Memory : Memory  X0=200
  Saturation : Saturate  UpperLimit=1  LowerLimit=-1  OutDataType=fixdt(1, 16)  OutScaling=2^0
  Saturation1 : Saturate  UpperLimit=1.01  LowerLimit=0.1  OutDataType=fixdt(1, 16)  OutScaling=2^0
  Subsystem : Subsystem
  Subsystem1 : Subsystem
  Subsystem2 : Subsystem
  Subsystem3 : Subsystem
  Sum : Sum  Inputs=|++  OutDataType=fixdt(1, 16)  OutScaling=2^0
  Sum10 : Sum  Inputs=++|  OutDataType=fixdt(1, 16)  OutScaling=2^0
  Sum2 : Sum  Inputs=|++  OutDataType=fixdt(1, 16)  OutScaling=2^0
  Sum{3..4,7..8} (4 alike) : Sum  Inputs=|+-  OutDataType=fixdt(1, 16)  OutScaling=2^0
  Sum5 : Sum  Inputs=|++  OutDataType=fixdt(1, 16)  OutScaling=2^0
  Sum6 : Sum  Inputs=+|+|+  OutDataType=fixdt(1, 16)  OutScaling=2^0
  Sum9 : Sum  Inputs=|+-+  OutDataType=fixdt(1, 16)  OutScaling=2^0
  Switch : Switch  Threshold=200*0.3  OutDataType=fixdt(1, 16)  OutScaling=2^0
  Switch1 : Switch  Threshold=99.999999  OutDataType=fixdt(1, 16)  OutScaling=2^0
  Switch2 : Switch  Threshold=99.999999  OutDataType=fixdt(1, 16)  OutScaling=2^0
  Switch3 : Switch  OutDataType=fixdt(1, 16)  OutScaling=2^0
  Transfer Fcn1 : TransferFcn  Numerator=1  Denominator=[1/(10) 1]
  Transport Delay : TransportDelay  DelayTime=2
  Transport Delay1 : TransportDelay  DelayTime=2
  ain1 : Gain  Gain=0.25  ParameterDataType=fixdt(1, 16)  ParameterScaling=2^0  OutDataType=fixdt(1, 16)  OutScaling=2^0
  ain2 : Gain  Gain=1/700  ParameterDataType=fixdt(1, 16)  ParameterScaling=2^0  OutDataType=fixdt(1, 16)  OutScaling=2^0
  ain3 : Gain  Gain=1/16.5  ParameterDataType=fixdt(1, 16)  ParameterScaling=2^0  OutDataType=fixdt(1, 16)  OutScaling=2^0
  ain4 : Gain  Gain=700  ParameterDataType=fixdt(1, 16)  ParameterScaling=2^0  OutDataType=fixdt(1, 16)  OutScaling=2^0
  ain5 : Gain  Gain=0.75  ParameterDataType=fixdt(1, 16)  ParameterScaling=2^0  OutDataType=fixdt(1, 16)  OutScaling=2^0
  ain6 : Gain  Gain=16.5  ParameterDataType=fixdt(1, 16)  ParameterScaling=2^0  OutDataType=fixdt(1, 16)  OutScaling=2^0
  ain7 : Gain  Gain=0.03  ParameterDataType=fixdt(1, 16)  ParameterScaling=2^0  OutDataType=fixdt(1, 16)  OutScaling=2^0
  ain8 : Gain  Gain=7  ParameterDataType=fixdt(1, 16)  ParameterScaling=2^0  OutDataType=fixdt(1, 16)  OutScaling=2^0
  ain9 : Gain  Gain=.3  ParameterDataType=fixdt(1, 16)  ParameterScaling=2^0  OutDataType=fixdt(1, 16)  OutScaling=2^0
  tag scope: Ibrefv14=global, boostv14=global, buckv14=global
  wires:
  Ibref-SUIM/1 -> ain9/1, ain8/1
  Switch/1 -> Transfer Fcn1/1
  ain9/1 -> Switch/3
  ain8/1 -> Switch/1
  [VbSUIMv14] -> Switch/2
  Saturation1/1 -> Switch1/1
  Transport Delay/1 -> Switch1/2
  [socv14] -> Transport Delay/1
  Memory/1 -> Switch2/1
  Switch2/1 -> Memory/1, Add1/1
  Gain2/1 -> Integrator/1
  Integrator/1 -> Add/1
  Gain1/1 -> Add/2
  Add/1 -> Saturation1/1
  Transport Delay1/1 -> Switch2/2
  [socv14] -> Transport Delay1/1
  [VbSUIMv14] -> Switch2/3
  Add1/1 -> Gain2/1, Gain1/1
  [VbSUIMv14] -> Add1/2
  [tv14] -> Subsystem/Enable
  Sum4/1 -> ain1/1, Subsystem2/1(In1)
  ain2/1 -> Saturation/1
  Subsystem2/1(Out1) -> Sum2/1
  ain1/1 -> Sum2/2
  Saturation/1 -> ain4/1, Switch1/3, Switch3/3, Switch3/2
  ain4/1 -> Sum3/1
  Sum3/1 -> ain3/1
  Subsystem1/1(Out1) -> Sum6/2
  ain5/1 -> Sum6/3
  Sum7/1 -> ain5/1, Subsystem1/1(In1)
  Sum2/1 -> Sum5/1
  Sum5/1 -> Sum8/1
  Sum8/1 -> ain6/1, Sum10/2
  Subsystem3/1(Out1) -> Sum/1
  ain6/1 -> Sum/2
  Sum/1 -> Sum9/1
  Sum9/1 -> Sum3/2, ain2/1
  ain3/1 -> Sum10/1
  ain7/1 -> Sum9/2
  Sum6/1 -> Sum4/1
  Sum10/1 -> Subsystem3/1(In1)
  [VcSUIMv14] -> Sum4/2
  [VcSUIMv14] -> Sum9/3
  [IbSUIMv14] -> Sum7/2
  [IbSUIMv14] -> Sum5/2
  [VbSUIMv14] -> Sum6/1
  [ISUIMv14] -> ain7/1
  [ISUIMv14] -> Sum8/2
  Subsystem/2(Out2) -> [boostv14]
  Subsystem/1(Out1) -> [buckv14]
  Transfer Fcn1/1 -> [Ibrefv14], Sum7/1
  Switch1/1 -> Switch3/1
  Switch3/1 -> Subsystem/1(In1)

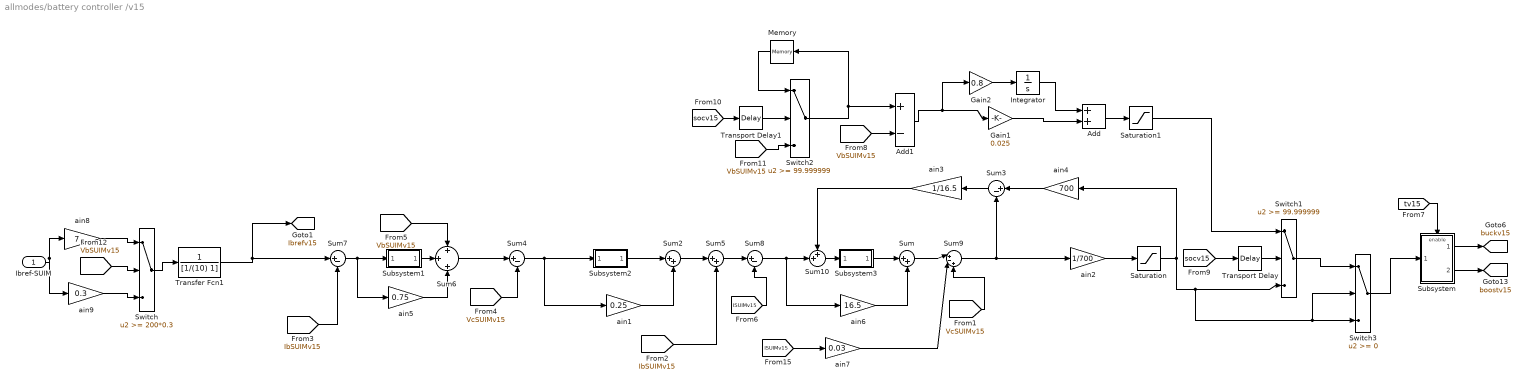
== system allmodes/battery controller /v15 ==
  Ibref-SUIM : Inport
  Add : Sum  OutDataType=fixdt(1, 16)  OutScaling=2^-10
  Add1 : Sum  Inputs=+-  OutDataType=fixdt(1, 16)  OutScaling=2^-10
  Gain1 : Gain  Gain=0.025  ParameterDataType=fixdt(1, 16)  ParameterScaling=2^0  OutDataType=fixdt(1, 16)  OutScaling=2^0
  Gain2 : Gain  Gain=0.8  ParameterDataType=fixdt(1, 16)  ParameterScaling=2^0  OutDataType=fixdt(1, 16)  OutScaling=2^0
  Integrator : Integrator
  Memory : Memory  X0=200
  Saturation : Saturate  UpperLimit=1  LowerLimit=-1  OutDataType=fixdt(1, 16)  OutScaling=2^0
  Saturation1 : Saturate  UpperLimit=1.01  LowerLimit=0.1  OutDataType=fixdt(1, 16)  OutScaling=2^0
  Subsystem : Subsystem
  Subsystem1 : Subsystem
  Subsystem2 : Subsystem
  Subsystem3 : Subsystem
  Sum : Sum  Inputs=|++  OutDataType=fixdt(1, 16)  OutScaling=2^0
  Sum10 : Sum  Inputs=++|  OutDataType=fixdt(1, 16)  OutScaling=2^0
  Sum2 : Sum  Inputs=|++  OutDataType=fixdt(1, 16)  OutScaling=2^0
  Sum{3..4,7..8} (4 alike) : Sum  Inputs=|+-  OutDataType=fixdt(1, 16)  OutScaling=2^0
  Sum5 : Sum  Inputs=|++  OutDataType=fixdt(1, 16)  OutScaling=2^0
  Sum6 : Sum  Inputs=+|+|+  OutDataType=fixdt(1, 16)  OutScaling=2^0
  Sum9 : Sum  Inputs=|+-+  OutDataType=fixdt(1, 16)  OutScaling=2^0
  Switch : Switch  Threshold=200*0.3  OutDataType=fixdt(1, 16)  OutScaling=2^0
  Switch1 : Switch  Threshold=99.999999  OutDataType=fixdt(1, 16)  OutScaling=2^0
  Switch2 : Switch  Threshold=99.999999  OutDataType=fixdt(1, 16)  OutScaling=2^0
  Switch3 : Switch  OutDataType=fixdt(1, 16)  OutScaling=2^0
  Transfer Fcn1 : TransferFcn  Numerator=1  Denominator=[1/(10) 1]
  Transport Delay : TransportDelay  DelayTime=2
  Transport Delay1 : TransportDelay  DelayTime=2
  ain1 : Gain  Gain=0.25  ParameterDataType=fixdt(1, 16)  ParameterScaling=2^0  OutDataType=fixdt(1, 16)  OutScaling=2^0
  ain2 : Gain  Gain=1/700  ParameterDataType=fixdt(1, 16)  ParameterScaling=2^0  OutDataType=fixdt(1, 16)  OutScaling=2^0
  ain3 : Gain  Gain=1/16.5  ParameterDataType=fixdt(1, 16)  ParameterScaling=2^0  OutDataType=fixdt(1, 16)  OutScaling=2^0
  ain4 : Gain  Gain=700  ParameterDataType=fixdt(1, 16)  ParameterScaling=2^0  OutDataType=fixdt(1, 16)  OutScaling=2^0
  ain5 : Gain  Gain=0.75  ParameterDataType=fixdt(1, 16)  ParameterScaling=2^0  OutDataType=fixdt(1, 16)  OutScaling=2^0
  ain6 : Gain  Gain=16.5  ParameterDataType=fixdt(1, 16)  ParameterScaling=2^0  OutDataType=fixdt(1, 16)  OutScaling=2^0
  ain7 : Gain  Gain=0.03  ParameterDataType=fixdt(1, 16)  ParameterScaling=2^0  OutDataType=fixdt(1, 16)  OutScaling=2^0
  ain8 : Gain  Gain=7  ParameterDataType=fixdt(1, 16)  ParameterScaling=2^0  OutDataType=fixdt(1, 16)  OutScaling=2^0
  ain9 : Gain  Gain=0.3  ParameterDataType=fixdt(1, 16)  ParameterScaling=2^0  OutDataType=fixdt(1, 16)  OutScaling=2^0
  tag scope: Ibrefv15=global, boostv15=global, buckv15=global
  wires:
  Ibref-SUIM/1 -> ain9/1, ain8/1
  Switch/1 -> Transfer Fcn1/1
  ain9/1 -> Switch/3
  ain8/1 -> Switch/1
  [VbSUIMv15] -> Switch/2
  Saturation1/1 -> Switch1/1
  Transport Delay/1 -> Switch1/2
  [socv15] -> Transport Delay/1
  Memory/1 -> Switch2/1
  Switch2/1 -> Memory/1, Add1/1
  Gain2/1 -> Integrator/1
  Integrator/1 -> Add/1
  Gain1/1 -> Add/2
  Add/1 -> Saturation1/1
  Transport Delay1/1 -> Switch2/2
  [socv15] -> Transport Delay1/1
  [VbSUIMv15] -> Switch2/3
  Add1/1 -> Gain2/1, Gain1/1
  [VbSUIMv15] -> Add1/2
  [tv15] -> Subsystem/Enable
  Sum4/1 -> ain1/1, Subsystem2/1(In1)
  ain2/1 -> Saturation/1
  Subsystem2/1(Out1) -> Sum2/1
  ain1/1 -> Sum2/2
  Saturation/1 -> ain4/1, Switch1/3, Switch3/3, Switch3/2
  ain4/1 -> Sum3/1
  Sum3/1 -> ain3/1
  Subsystem1/1(Out1) -> Sum6/2
  ain5/1 -> Sum6/3
  Sum7/1 -> ain5/1, Subsystem1/1(In1)
  Sum2/1 -> Sum5/1
  Sum5/1 -> Sum8/1
  Sum8/1 -> ain6/1, Sum10/2
  Subsystem3/1(Out1) -> Sum/1
  ain6/1 -> Sum/2
  Sum/1 -> Sum9/1
  Sum9/1 -> Sum3/2, ain2/1
  ain3/1 -> Sum10/1
  ain7/1 -> Sum9/2
  Sum6/1 -> Sum4/1
  Sum10/1 -> Subsystem3/1(In1)
  [VcSUIMv15] -> Sum4/2
  [VcSUIMv15] -> Sum9/3
  [IbSUIMv15] -> Sum7/2
  [IbSUIMv15] -> Sum5/2
  [VbSUIMv15] -> Sum6/1
  [ISUIMv15] -> ain7/1
  [ISUIMv15] -> Sum8/2
  Subsystem/2(Out2) -> [boostv15]
  Subsystem/1(Out1) -> [buckv15]
  Transfer Fcn1/1 -> [Ibrefv15], Sum7/1
  Switch1/1 -> Switch3/1
  Switch3/1 -> Subsystem/1(In1)

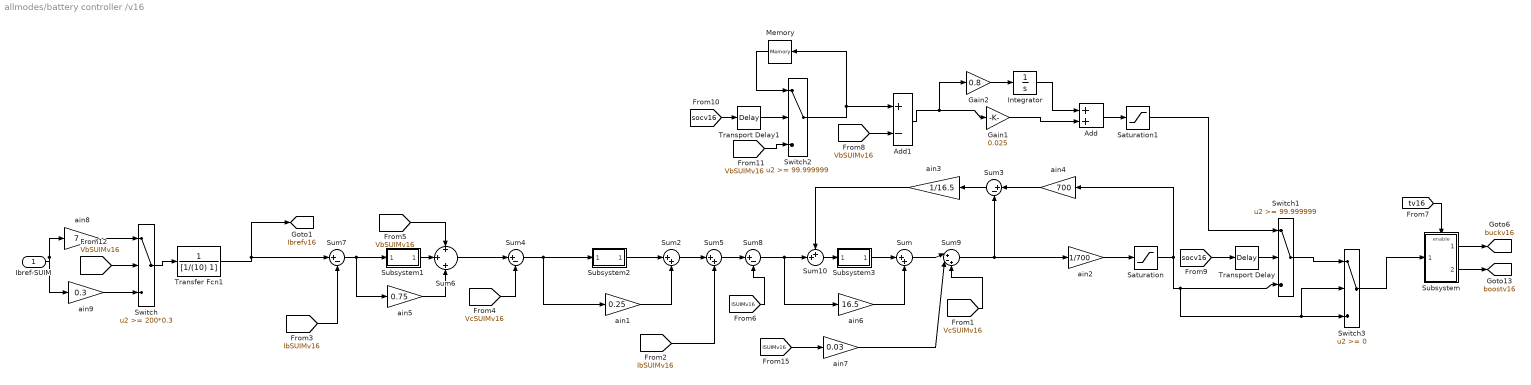
== system allmodes/battery controller /v16 ==
  Ibref-SUIM : Inport
  Add : Sum  OutDataType=fixdt(1, 16)  OutScaling=2^-10
  Add1 : Sum  Inputs=+-  OutDataType=fixdt(1, 16)  OutScaling=2^-10
  Gain1 : Gain  Gain=0.025  ParameterDataType=fixdt(1, 16)  ParameterScaling=2^0  OutDataType=fixdt(1, 16)  OutScaling=2^0
  Gain2 : Gain  Gain=0.8  ParameterDataType=fixdt(1, 16)  ParameterScaling=2^0  OutDataType=fixdt(1, 16)  OutScaling=2^0
  Integrator : Integrator
  Memory : Memory  X0=200
  Saturation : Saturate  UpperLimit=1  LowerLimit=-1  OutDataType=fixdt(1, 16)  OutScaling=2^0
  Saturation1 : Saturate  UpperLimit=1.01  LowerLimit=0.1  OutDataType=fixdt(1, 16)  OutScaling=2^0
  Subsystem : Subsystem
  Subsystem1 : Subsystem
  Subsystem2 : Subsystem
  Subsystem3 : Subsystem
  Sum : Sum  Inputs=|++  OutDataType=fixdt(1, 16)  OutScaling=2^0
  Sum10 : Sum  Inputs=++|  OutDataType=fixdt(1, 16)  OutScaling=2^0
  Sum2 : Sum  Inputs=|++  OutDataType=fixdt(1, 16)  OutScaling=2^0
  Sum{3..4,7..8} (4 alike) : Sum  Inputs=|+-  OutDataType=fixdt(1, 16)  OutScaling=2^0
  Sum5 : Sum  Inputs=|++  OutDataType=fixdt(1, 16)  OutScaling=2^0
  Sum6 : Sum  Inputs=+|+|+  OutDataType=fixdt(1, 16)  OutScaling=2^0
  Sum9 : Sum  Inputs=|+-+  OutDataType=fixdt(1, 16)  OutScaling=2^0
  Switch : Switch  Threshold=200*0.3  OutDataType=fixdt(1, 16)  OutScaling=2^0
  Switch1 : Switch  Threshold=99.999999  OutDataType=fixdt(1, 16)  OutScaling=2^0
  Switch2 : Switch  Threshold=99.999999  OutDataType=fixdt(1, 16)  OutScaling=2^0
  Switch3 : Switch  OutDataType=fixdt(1, 16)  OutScaling=2^0
  Transfer Fcn1 : TransferFcn  Numerator=1  Denominator=[1/(10) 1]
  Transport Delay : TransportDelay  DelayTime=2
  Transport Delay1 : TransportDelay  DelayTime=2
  ain1 : Gain  Gain=0.25  ParameterDataType=fixdt(1, 16)  ParameterScaling=2^0  OutDataType=fixdt(1, 16)  OutScaling=2^0
  ain2 : Gain  Gain=1/700  ParameterDataType=fixdt(1, 16)  ParameterScaling=2^0  OutDataType=fixdt(1, 16)  OutScaling=2^0
  ain3 : Gain  Gain=1/16.5  ParameterDataType=fixdt(1, 16)  ParameterScaling=2^0  OutDataType=fixdt(1, 16)  OutScaling=2^0
  ain4 : Gain  Gain=700  ParameterDataType=fixdt(1, 16)  ParameterScaling=2^0  OutDataType=fixdt(1, 16)  OutScaling=2^0
  ain5 : Gain  Gain=0.75  ParameterDataType=fixdt(1, 16)  ParameterScaling=2^0  OutDataType=fixdt(1, 16)  OutScaling=2^0
  ain6 : Gain  Gain=16.5  ParameterDataType=fixdt(1, 16)  ParameterScaling=2^0  OutDataType=fixdt(1, 16)  OutScaling=2^0
  ain7 : Gain  Gain=0.03  ParameterDataType=fixdt(1, 16)  ParameterScaling=2^0  OutDataType=fixdt(1, 16)  OutScaling=2^0
  ain8 : Gain  Gain=7  ParameterDataType=fixdt(1, 16)  ParameterScaling=2^0  OutDataType=fixdt(1, 16)  OutScaling=2^0
  ain9 : Gain  Gain=0.3  ParameterDataType=fixdt(1, 16)  ParameterScaling=2^0  OutDataType=fixdt(1, 16)  OutScaling=2^0
  tag scope: Ibrefv16=global, boostv16=global, buckv16=global
  wires:
  Ibref-SUIM/1 -> ain9/1, ain8/1
  Switch/1 -> Transfer Fcn1/1
  ain9/1 -> Switch/3
  ain8/1 -> Switch/1
  [VbSUIMv16] -> Switch/2
  Saturation1/1 -> Switch1/1
  Transport Delay/1 -> Switch1/2
  [socv16] -> Transport Delay/1
  Memory/1 -> Switch2/1
  Switch2/1 -> Memory/1, Add1/1
  Gain2/1 -> Integrator/1
  Integrator/1 -> Add/1
  Gain1/1 -> Add/2
  Add/1 -> Saturation1/1
  Transport Delay1/1 -> Switch2/2
  [socv16] -> Transport Delay1/1
  [VbSUIMv16] -> Switch2/3
  Add1/1 -> Gain2/1, Gain1/1
  [VbSUIMv16] -> Add1/2
  [tv16] -> Subsystem/Enable
  Sum4/1 -> ain1/1, Subsystem2/1(In1)
  ain2/1 -> Saturation/1
  Subsystem2/1(Out1) -> Sum2/1
  ain1/1 -> Sum2/2
  Saturation/1 -> ain4/1, Switch1/3, Switch3/3, Switch3/2
  ain4/1 -> Sum3/1
  Sum3/1 -> ain3/1
  Subsystem1/1(Out1) -> Sum6/2
  ain5/1 -> Sum6/3
  Sum7/1 -> ain5/1, Subsystem1/1(In1)
  Sum2/1 -> Sum5/1
  Sum5/1 -> Sum8/1
  Sum8/1 -> ain6/1, Sum10/2
  Subsystem3/1(Out1) -> Sum/1
  ain6/1 -> Sum/2
  Sum/1 -> Sum9/1
  Sum9/1 -> Sum3/2, ain2/1
  ain3/1 -> Sum10/1
  ain7/1 -> Sum9/2
  Sum6/1 -> Sum4/1
  Sum10/1 -> Subsystem3/1(In1)
  [VcSUIMv16] -> Sum4/2
  [VcSUIMv16] -> Sum9/3
  [IbSUIMv16] -> Sum7/2
  [IbSUIMv16] -> Sum5/2
  [VbSUIMv16] -> Sum6/1
  [ISUIMv16] -> ain7/1
  [ISUIMv16] -> Sum8/2
  Subsystem/2(Out2) -> [boostv16]
  Subsystem/1(Out1) -> [buckv16]
  Transfer Fcn1/1 -> [Ibrefv16], Sum7/1
  Switch1/1 -> Switch3/1
  Switch3/1 -> Subsystem/1(In1)

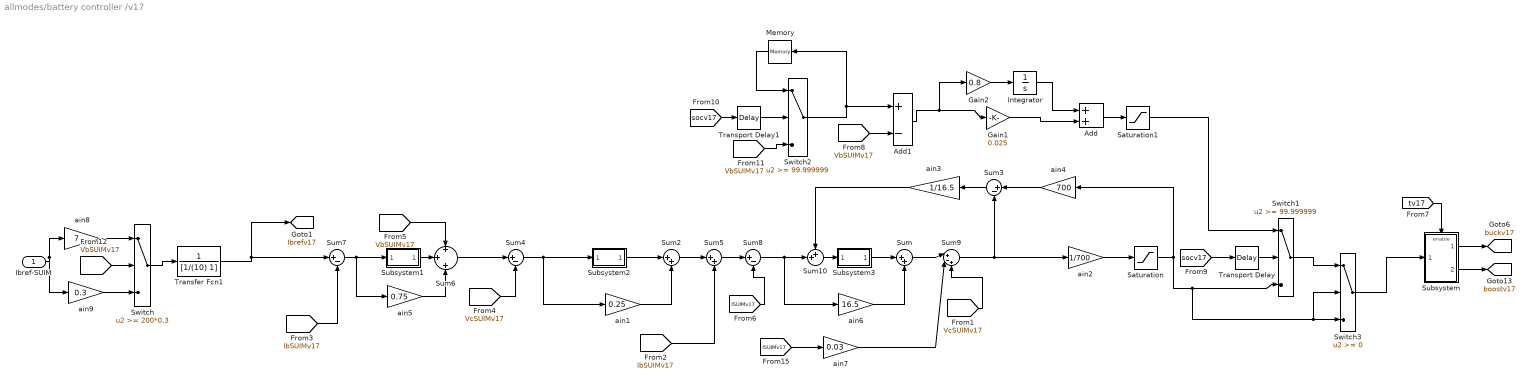
== system allmodes/battery controller /v17 ==
  Ibref-SUIM : Inport
  Add : Sum  OutDataType=fixdt(1, 16)  OutScaling=2^-10
  Add1 : Sum  Inputs=+-  OutDataType=fixdt(1, 16)  OutScaling=2^-10
  Gain1 : Gain  Gain=0.025  ParameterDataType=fixdt(1, 16)  ParameterScaling=2^0  OutDataType=fixdt(1, 16)  OutScaling=2^0
  Gain2 : Gain  Gain=0.8  ParameterDataType=fixdt(1, 16)  ParameterScaling=2^0  OutDataType=fixdt(1, 16)  OutScaling=2^0
  Integrator : Integrator
  Memory : Memory  X0=200
  Saturation : Saturate  UpperLimit=1  LowerLimit=-1  OutDataType=fixdt(1, 16)  OutScaling=2^0
  Saturation1 : Saturate  UpperLimit=1.01  LowerLimit=0.1  OutDataType=fixdt(1, 16)  OutScaling=2^0
  Subsystem : Subsystem
  Subsystem1 : Subsystem
  Subsystem2 : Subsystem
  Subsystem3 : Subsystem
  Sum : Sum  Inputs=|++  OutDataType=fixdt(1, 16)  OutScaling=2^0
  Sum10 : Sum  Inputs=++|  OutDataType=fixdt(1, 16)  OutScaling=2^0
  Sum2 : Sum  Inputs=|++  OutDataType=fixdt(1, 16)  OutScaling=2^0
  Sum{3..4,7..8} (4 alike) : Sum  Inputs=|+-  OutDataType=fixdt(1, 16)  OutScaling=2^0
  Sum5 : Sum  Inputs=|++  OutDataType=fixdt(1, 16)  OutScaling=2^0
  Sum6 : Sum  Inputs=+|+|+  OutDataType=fixdt(1, 16)  OutScaling=2^0
  Sum9 : Sum  Inputs=|+-+  OutDataType=fixdt(1, 16)  OutScaling=2^0
  Switch : Switch  Threshold=200*0.3  OutDataType=fixdt(1, 16)  OutScaling=2^0
  Switch1 : Switch  Threshold=99.999999  OutDataType=fixdt(1, 16)  OutScaling=2^0
  Switch2 : Switch  Threshold=99.999999  OutDataType=fixdt(1, 16)  OutScaling=2^0
  Switch3 : Switch  OutDataType=fixdt(1, 16)  OutScaling=2^0
  Transfer Fcn1 : TransferFcn  Numerator=1  Denominator=[1/(10) 1]
  Transport Delay : TransportDelay  DelayTime=2
  Transport Delay1 : TransportDelay  DelayTime=2
  ain1 : Gain  Gain=0.25  ParameterDataType=fixdt(1, 16)  ParameterScaling=2^0  OutDataType=fixdt(1, 16)  OutScaling=2^0
  ain2 : Gain  Gain=1/700  ParameterDataType=fixdt(1, 16)  ParameterScaling=2^0  OutDataType=fixdt(1, 16)  OutScaling=2^0
  ain3 : Gain  Gain=1/16.5  ParameterDataType=fixdt(1, 16)  ParameterScaling=2^0  OutDataType=fixdt(1, 16)  OutScaling=2^0
  ain4 : Gain  Gain=700  ParameterDataType=fixdt(1, 16)  ParameterScaling=2^0  OutDataType=fixdt(1, 16)  OutScaling=2^0
  ain5 : Gain  Gain=0.75  ParameterDataType=fixdt(1, 16)  ParameterScaling=2^0  OutDataType=fixdt(1, 16)  OutScaling=2^0
  ain6 : Gain  Gain=16.5  ParameterDataType=fixdt(1, 16)  ParameterScaling=2^0  OutDataType=fixdt(1, 16)  OutScaling=2^0
  ain7 : Gain  Gain=0.03  ParameterDataType=fixdt(1, 16)  ParameterScaling=2^0  OutDataType=fixdt(1, 16)  OutScaling=2^0
  ain8 : Gain  Gain=7  ParameterDataType=fixdt(1, 16)  ParameterScaling=2^0  OutDataType=fixdt(1, 16)  OutScaling=2^0
  ain9 : Gain  Gain=0.3  ParameterDataType=fixdt(1, 16)  ParameterScaling=2^0  OutDataType=fixdt(1, 16)  OutScaling=2^0
  tag scope: Ibrefv17=global, boostv17=global, buckv17=global
  wires:
  Ibref-SUIM/1 -> ain9/1, ain8/1
  Switch/1 -> Transfer Fcn1/1
  ain9/1 -> Switch/3
  ain8/1 -> Switch/1
  [VbSUIMv17] -> Switch/2
  Saturation1/1 -> Switch1/1
  Transport Delay/1 -> Switch1/2
  [socv17] -> Transport Delay/1
  Memory/1 -> Switch2/1
  Switch2/1 -> Memory/1, Add1/1
  Gain2/1 -> Integrator/1
  Integrator/1 -> Add/1
  Gain1/1 -> Add/2
  Add/1 -> Saturation1/1
  Transport Delay1/1 -> Switch2/2
  [socv17] -> Transport Delay1/1
  [VbSUIMv17] -> Switch2/3
  Add1/1 -> Gain2/1, Gain1/1
  [VbSUIMv17] -> Add1/2
  [tv17] -> Subsystem/Enable
  Sum4/1 -> ain1/1, Subsystem2/1(In1)
  ain2/1 -> Saturation/1
  Subsystem2/1(Out1) -> Sum2/1
  ain1/1 -> Sum2/2
  Saturation/1 -> ain4/1, Switch1/3, Switch3/3, Switch3/2
  ain4/1 -> Sum3/1
  Sum3/1 -> ain3/1
  Subsystem1/1(Out1) -> Sum6/2
  ain5/1 -> Sum6/3
  Sum7/1 -> ain5/1, Subsystem1/1(In1)
  Sum2/1 -> Sum5/1
  Sum5/1 -> Sum8/1
  Sum8/1 -> ain6/1, Sum10/2
  Subsystem3/1(Out1) -> Sum/1
  ain6/1 -> Sum/2
  Sum/1 -> Sum9/1
  Sum9/1 -> Sum3/2, ain2/1
  ain3/1 -> Sum10/1
  ain7/1 -> Sum9/2
  Sum6/1 -> Sum4/1
  Sum10/1 -> Subsystem3/1(In1)
  [VcSUIMv17] -> Sum4/2
  [VcSUIMv17] -> Sum9/3
  [IbSUIMv17] -> Sum7/2
  [IbSUIMv17] -> Sum5/2
  [VbSUIMv17] -> Sum6/1
  [ISUIMv17] -> ain7/1
  [ISUIMv17] -> Sum8/2
  Subsystem/2(Out2) -> [boostv17]
  Subsystem/1(Out1) -> [buckv17]
  Transfer Fcn1/1 -> [Ibrefv17], Sum7/1
  Switch1/1 -> Switch3/1
  Switch3/1 -> Subsystem/1(In1)
